simulink model "GSK_PVModel_03"  (R2016a)
settings: Solver=FixedStepAuto  StartTime=0.0  StopTime=10.0  FixedStep=0.0001  RelTol=1e-3
values from neighbouring files (symbols this model uses):
  a = 1.5    [GSK_PVModelValues.m]    (also in GSK_PVModelValues_05.m)
  G_n = 1000    [GSK_PVModelValues.m]    (also in GSK_PVModelValues_05.m)
  I_pv_n = 6.5    [GSK_PVModelValues.m]    (also in GSK_PVModelValues_05.m)
  I_sc_n = 6.43    [GSK_PVModelValues.m]    (also in GSK_PVModelValues_05.m)
  K_I = 3.5e-3    (= 0.0035)    [GSK_PVModelValues.m]    (also in GSK_PVModelValues_05.m)
  K_V = - 235.5e-3    (= -0.2355)    [GSK_PVModelValues.m]    (also in GSK_PVModelValues_05.m)
  R_p = 1000    [GSK_PVModelValues.m]    (also in GSK_PVModelValues_05.m)
  R_s = 1e-3*128    (= 0.128)    [GSK_PVModelValues.m]    (also in GSK_PVModelValues_05.m)
  T = 273+40    (= 313)    [GSK_PVModelValues.m]    (also in GSK_PVModelValues_05.m)
  T_n = 25+273    (= 298)    [GSK_PVModelValues.m]    (also in GSK_PVModelValues_05.m)
  V_oc_n = 85.6    [GSK_PVModelValues.m]    (also in GSK_PVModelValues_05.m)
  V_t = N_s*k/q*T    [GSK_PVModelValues_05.m]
libraries: fl_lib x11, nesl_utility x5, simulink x3
settings Model: Creator=gadis  LastModifiedBy=gadis

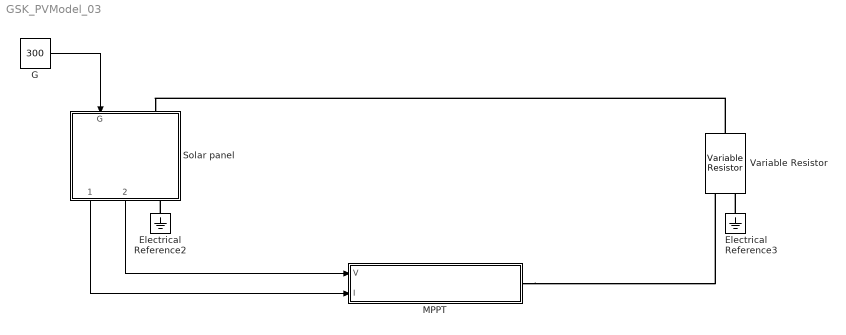
== system GSK_PVModel_03 ==
  Electrical Reference2 : fl_lib/Electrical/Electrical Elements/Electrical Reference
  Electrical Reference3 : fl_lib/Electrical/Electrical Elements/Electrical Reference
  G : Constant  Value=300
  MPPT : Subsystem
  Solar panel : Subsystem
  Variable Resistor : fl_lib/Electrical/Electrical Elements/Variable Resistor  Rmin=0.01 Ohm  i_specify=off  i_priority=None  i=0 A  v_specify=off  v_priority=None  v=0 V
  wires:
  Solar panel/2(V Simulink) -> MPPT/1(V)
  Solar panel/1(I Simulink) -> MPPT/2(I)
  G/1 -> Solar panel/1(G)
  connections:
  Electrical Reference3/LConn1 -- Variable Resistor/LConn2
  Variable Resistor/RConn1 -- Solar panel/LConn1
  Electrical Reference2/LConn1 -- Solar panel/RConn1
  MPPT/RConn1 -- Variable Resistor/LConn1

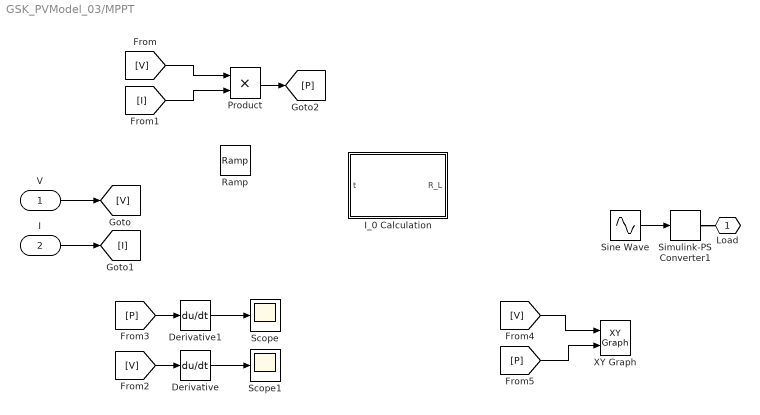
== system GSK_PVModel_03/MPPT ==
  V : Inport
  I : Inport  Port=2
  Derivative : Derivative
  Derivative1 : Derivative
  I_0 Calculation : MATLAB Function  TreatAsAtomicUnit=on
  Product : Product
  Ramp : simulink/Sources/Ramp  slope=1  start=0  X0=0
  Scope : Scope
  Scope1 : Scope
  Simulink-PS Converter1 : nesl_utility/Simulink-PS Converter  PhysicalDomain=network_engine_domain  SubClassName=ps_input  LeftPortType=input  RightPortType=output  PseudoPeriodic=off  Frequencies=[]  NoiseDistribution=none  NoiseParameters=[]  Unit=1  AffineConversion=off  InputFiltering=off  SimscapeFilterOrder=1  InputFilterTimeConstant=0.001  UdotUserProvided=1
  Sine Wave : Sin  Amplitude=25  Bias=25  SampleTime=0
  XY Graph : simulink/Sinks/XY Graph  xmin=-1  xmax=100  ymin=-1  ymax=500  st=-1
  Load : PMIOPort  Port=1  Side=Right
  wires:
  Sine Wave/1 -> Simulink-PS Converter1/1
  V/1 -> [V]
  I/1 -> [I]
  [I] -> Product/2
  [V] -> Product/1
  Product/1 -> [P]
  [V] -> Derivative/1
  [P] -> Derivative1/1
  Derivative1/1 -> Scope/1
  Derivative/1 -> Scope1/1
  [V] -> XY Graph/1
  [P] -> XY Graph/2
  connections:
  Simulink-PS Converter1/RConn1 -- Load/RConn1

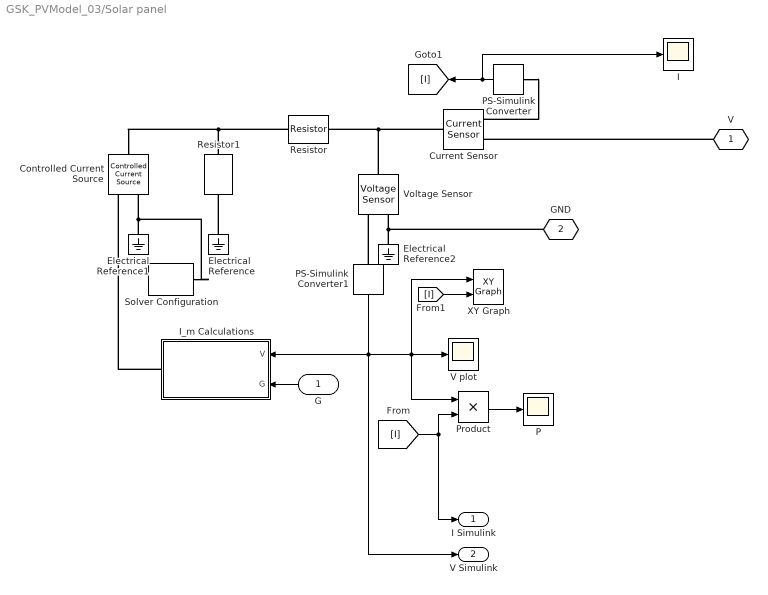
== system GSK_PVModel_03/Solar panel ==
  G : Inport
  Controlled Current Source : fl_lib/Electrical/Electrical Sources/Controlled Current Source
  Current Sensor : fl_lib/Electrical/Electrical Sensors/Current Sensor
  Electrical Reference : fl_lib/Electrical/Electrical Elements/Electrical Reference
  Electrical Reference1 : fl_lib/Electrical/Electrical Elements/Electrical Reference
  Electrical Reference2 : fl_lib/Electrical/Electrical Elements/Electrical Reference
  I : Scope
  I_m Calculations : Subsystem
  P : Scope
  PS-Simulink Converter : nesl_utility/PS-Simulink Converter  PhysicalDomain=network_engine_domain  SubClassName=ps_output  LeftPortType=input  RightPortType=output  PseudoPeriodic=off  Frequencies=[]  Unit=1  AffineConversion=off
  PS-Simulink Converter1 : nesl_utility/PS-Simulink Converter  PhysicalDomain=network_engine_domain  SubClassName=ps_output  LeftPortType=input  RightPortType=output  PseudoPeriodic=off  Frequencies=[]  Unit=1  AffineConversion=off
  Product : Product
  Resistor : fl_lib/Electrical/Electrical Elements/Resistor  R=R_s Ohm  i_specify=off  i_priority=None  i=0 A  v_specify=off  v_priority=None  v=0 V
  Resistor1 : fl_lib/Electrical/Electrical Elements/Resistor  R=R_p Ohm  i_specify=off  i_priority=None  i=0 A  v_specify=off  v_priority=None  v=0 V
  Solver Configuration : nesl_utility/Solver Configuration  PhysicalDomain=network_engine_domain  SubClassName=solver  LeftPortType=input  RightPortType=generic  Accelerate=off  Tones=[]  Harmonics=[]  SimulateNoise=off  Profile=off  UseLocalSampling=off  EnableSwitchedLinearOptims=on  FrequencyDomain=off  UseCCode=off  RelTol=0.001  AbsTol=1e-06  MinStep=1e-09  ToWorkspace=off  RevertToSquareIcSolve=off  NumHomotopyIterations=100  PhasorMode=off  PhasorModeNumHarmonics=1  OverrideAbsTol=off  DoDC=off  ResidualTolerance=1e-09  UseLocalSolver=off  LocalSolverChoice=NE_BACKWARD_EULER_ADVANCER  LocalSolverSampleTime=0.001  DoFixedCost=off  MaxNonlinIter=3  MaxModeIter=2  LinearAlgebra=Sparse  DelaysMemoryBudget=1024  AutomaticFiltering=on  FilteringTimeConstant=0.001
  V plot : Scope
  Voltage Sensor : fl_lib/Electrical/Electrical Sensors/Voltage Sensor
  XY Graph : simulink/Sinks/XY Graph  xmin=-1  xmax=100  ymin=-1  ymax=0010  st=-1
  V : PMIOPort  Port=1  Side=Left
  GND : PMIOPort  Port=2  Side=Right
  I Simulink : Outport
  V Simulink : Outport  Port=2
  wires:
  G/1 -> I_m Calculations/2(G)
  PS-Simulink Converter1/1 -> V Simulink/1, XY Graph/1, Product/1, V plot/1, I_m Calculations/1(V)
  PS-Simulink Converter/1 -> I/1, [I]
  [I] -> XY Graph/2
  Product/1 -> P/1
  [I] -> Product/2, I Simulink/1
  connections:
  V/RConn1 -- Current Sensor/RConn2
  Voltage Sensor/LConn1 -- Resistor/RConn1 -- Current Sensor/LConn1
  PS-Simulink Converter/LConn1 -- Current Sensor/RConn1
  Electrical Reference/LConn1 -- Resistor1/RConn1
  Resistor/LConn1 -- Resistor1/LConn1 -- Controlled Current Source/LConn1
  I_m Calculations/RConn1 -- Controlled Current Source/RConn1
  Electrical Reference2/LConn1 -- GND/RConn1 -- Voltage Sensor/RConn2
  Electrical Reference1/LConn1 -- Solver Configuration/RConn1 -- Controlled Current Source/RConn2
  PS-Simulink Converter1/LConn1 -- Voltage Sensor/RConn1

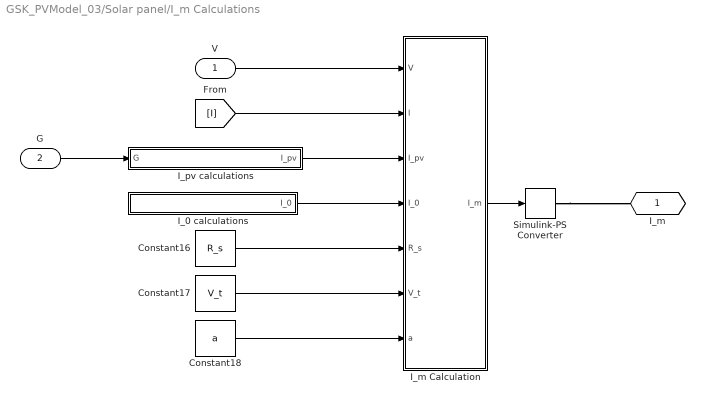
== system GSK_PVModel_03/Solar panel/I_m Calculations ==
  V : Inport
  G : Inport  Port=2
  Constant16 : Constant  Value=R_s
  Constant17 : Constant  Value=V_t
  Constant18 : Constant  Value=a
  I_0 calculations : Subsystem
  I_m Calculation : MATLAB Function  TreatAsAtomicUnit=on
  I_pv calculations : Subsystem
  Simulink-PS Converter : nesl_utility/Simulink-PS Converter  PhysicalDomain=network_engine_domain  SubClassName=ps_input  LeftPortType=input  RightPortType=output  PseudoPeriodic=off  Frequencies=[]  NoiseDistribution=none  NoiseParameters=[]  Unit=1  AffineConversion=off  InputFiltering=off  SimscapeFilterOrder=1  InputFilterTimeConstant=0.001  UdotUserProvided=1
  I_m : PMIOPort  Port=1  Side=Right
  wires:
  [I] -> I_m Calculation/2(I)
  V/1 -> I_m Calculation/1(V)
  I_m Calculation/1(I_m) -> Simulink-PS Converter/1
  I_pv calculations/1(I_pv) -> I_m Calculation/3(I_pv)
  G/1 -> I_pv calculations/1(G)
  I_0 calculations/1(I_0) -> I_m Calculation/4(I_0)
  Constant16/1 -> I_m Calculation/5(R_s)
  Constant18/1 -> I_m Calculation/7(a)
  Constant17/1 -> I_m Calculation/6(V_t)
  connections:
  Simulink-PS Converter/RConn1 -- I_m/RConn1

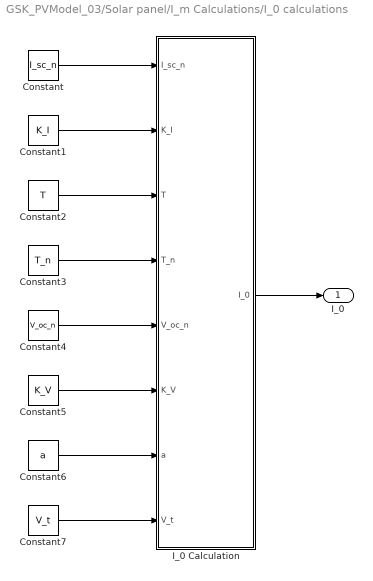
== system GSK_PVModel_03/Solar panel/I_m Calculations/I_0 calculations ==
  Constant : Constant  Value=I_sc_n
  Constant1 : Constant  Value=K_I
  Constant2 : Constant  Value=T
  Constant3 : Constant  Value=T_n
  Constant4 : Constant  Value=V_oc_n
  Constant5 : Constant  Value=K_V
  Constant6 : Constant  Value=a
  Constant7 : Constant  Value=V_t
  I_0 Calculation : MATLAB Function  TreatAsAtomicUnit=on
  I_0 : Outport
  wires:
  I_0 Calculation/1(I_0) -> I_0/1
  Constant7/1 -> I_0 Calculation/8(V_t)
  Constant5/1 -> I_0 Calculation/6(K_V)
  Constant4/1 -> I_0 Calculation/5(V_oc_n)
  Constant1/1 -> I_0 Calculation/2(K_I)
  Constant/1 -> I_0 Calculation/1(I_sc_n)
  Constant6/1 -> I_0 Calculation/7(a)
  Constant2/1 -> I_0 Calculation/3(T)
  Constant3/1 -> I_0 Calculation/4(T_n)

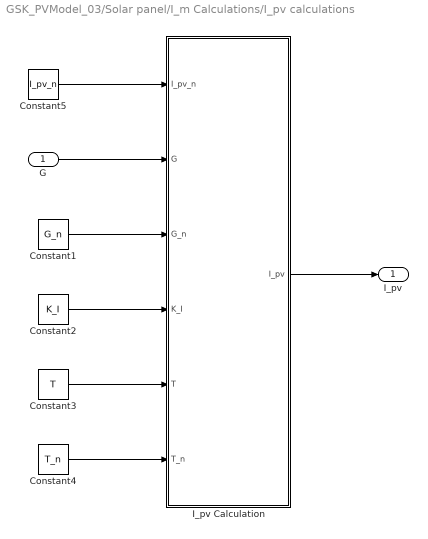
== system GSK_PVModel_03/Solar panel/I_m Calculations/I_pv calculations ==
  G : Inport
  Constant1 : Constant  Value=G_n
  Constant2 : Constant  Value=K_I
  Constant3 : Constant  Value=T
  Constant4 : Constant  Value=T_n
  Constant5 : Constant  Value=I_pv_n
  I_pv Calculation : MATLAB Function  TreatAsAtomicUnit=on
  I_pv : Outport
  wires:
  Constant5/1 -> I_pv Calculation/1(I_pv_n)
  G/1 -> I_pv Calculation/2(G)
  I_pv Calculation/1(I_pv) -> I_pv/1
  Constant1/1 -> I_pv Calculation/3(G_n)
  Constant2/1 -> I_pv Calculation/4(K_I)
  Constant3/1 -> I_pv Calculation/5(T)
  Constant4/1 -> I_pv Calculation/6(T_n)

== matlab function GSK_PVModel_03/Solar panel/I_m Calculations/I_pv calculations/I_pv Calculation ==
  data: I_pv_n input; I_pv output; G input; G_n input; K_I input; T input; T_n input
function I_pv = fcn(I_pv_n, G, G_n, K_I, T, T_n )
%#codegen
Delta_T = (T - T_n);
I_pv = (I_pv_n + K_I*Delta_T)*G/G_n;

== matlab function GSK_PVModel_03/Solar panel/I_m Calculations/I_0 calculations/I_0 Calculation ==
  data: I_sc_n input; K_I input; T input; T_n input; I_0 output; V_oc_n input; K_V input; a input; V_t input
function I_0 = fcn(I_sc_n, K_I, T, T_n, V_oc_n, K_V, a, V_t)
%#codegen
Delta_T = (T - T_n);
I_0 = (I_sc_n + K_I * Delta_T )/(exp((V_oc_n + K_V*Delta_T)/(a*V_t))-1);

== matlab function GSK_PVModel_03/Solar panel/I_m Calculations/I_m Calculation ==
  data: V input; I input; I_pv input; I_0 input; R_s input; V_t input; I_m output; a input
function I_m = fcn(V, I, I_pv, I_0, R_s, V_t, a)
%#codegen
I_m = I_pv - I_0*(exp((V+R_s*I)/(V_t*a)-1));

== matlab function GSK_PVModel_03/MPPT/I_0 Calculation ==
  data: t input; R_L output
function R_L = fcn(t)
%#codegen
R_L = mod(t,1);
